simulink model "feedback_linearization_2015"  (R2020a)
settings: Solver=ode4  StartTime=0.0  StopTime=inf  FixedStep=0.002  RelTol=1e-3  EnableMultiTasking=on
undefined symbols (not defined in the file): Afe, g, gains_increasing, K, Kp_i_increasing, L, m, m0, REG_linearization, Ti_i_increasing, x, x_eq_increasing, y
libraries: PoliArd x6, simulink x6
settings Model: ExtModeTrigDuration=2  Creator=User  LastModifiedBy=miche
settings DataIOCC: LimitDataPoints=on  SaveFormat=Array  ReturnWorkspaceOutputs=off
settings OptimizationCC: LifeSpan=1  EfficientTunableParamExpr=on
settings DebuggingCC: UnderspecifiedInitializationDetection=Classic  MergeDetectMultiDrivingBlocksExec=none  SFUnexpectedBacktrackingDiag=warning  SFNoUnconditionalDefaultTransitionDiag=warning  SFExecutionAtInitializationDiag=none  ArithmeticOperatorsInVariantConditions=warning
settings HardwareCC: ProdBitPerPointer=32  ProdBitPerSizeT=32  ProdBitPerPtrDiffT=32  ProdLargestAtomicInteger=Long  ProdLargestAtomicFloat=Double  ProdIntDivRoundTo=Undefined  ProdWordSize=32  ProdHWDeviceType=ARM Compatible->ARM Cortex
settings ModelReferenceCC: PropagateSignalLabelsOutOfModel=off
settings SFSimCC: SimUseLocalCustomCode=off  MATLABDynamicMemAlloc=off  CustomCodeUndefinedFunction=UseInterfaceOnly
settings RTWCC: Description=Run on Target Hardware  SystemTargetFile=realtime.tlc  GenerateMakefile=off  TemplateMakefile=realtime.tmf  RTWVerbose=off  RTWUseLocalCustomCode=off
settings CodeAppCC: StateflowObjectComments=on
settings STFCustomTargetCC: TargetLibSuffix=.a  GenerateSampleERTMain=on  ERTCustomFileBanners=on  SupportNonInlinedSFcns=off  RemoveResetFunc=on  SupportVariableSizeSignals=on  MATLABClassNameForMDSCustomization=Simulink.SoftwareTarget.ERTCustomization  SystemTargetFile=realtime.tlc
settings ERTTargetCC: MultiwordLength=2048  GenerateSampleERTMain=on  ParMdlRefBuildCompliant=off  CompOptLevelCompliant=off  ConcurrentExecutionCompliant=off  CombineOutputUpdateFcns=off  SupportContinuousTime=on  SupportVariableSizeSignals=on  ModelStepFunctionPrototypeControlCompliant=off  CPPClassGenCompliant=off  UseToolchainInfoCompliant=off  ExtModeTransport=3  ExtModeMexFile=ext_serial_win32_comm_rtt  ExtModeMexArgs=0 1 9600  ERTSrcFileBannerTemplate=realtime_code_template.cgt  ERTHdrFileBannerTemplate=realtime_code_template.cgt  ERTDataSrcFileTemplate=realtime_code_template.cgt  ERTDataHdrFileTemplate=realtime_code_template.cgt  ERTCustomFileTemplate=realtime_file_process.tlc  ConvertIfToSwitch=off  SuppressUnreachableDefaultCases=off
settings ConfigComp: CovMetricSettings=dw  CovSaveCumulativeToWorkspaceVar=on  CovSaveSingleToWorkspaceVar=on  CovExternalEMLEnable=off

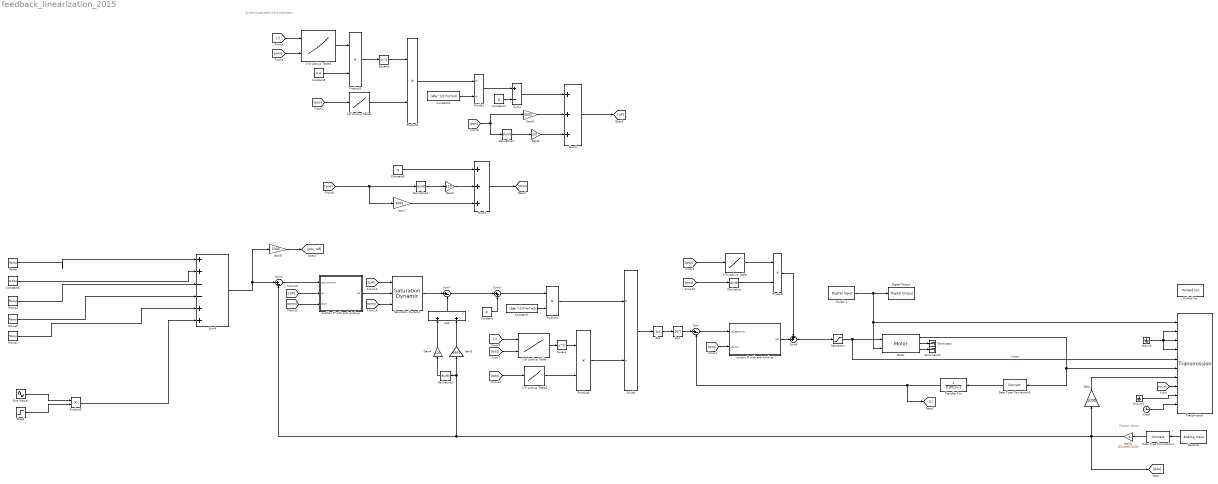
== system feedback_linearization_2015 ==
  note: Dynamic saturation limit estimation
  note: Position sensor
  1-D Lookup Table : Lookup_n-D  NumberOfTableDimensions=1  BreakpointsForDimension1=[0.0085 x_eq_increasing]  Table=[gains_increasing(1) gains_increasing]  InternalRulePriority=Speed  RndMeth=Simplest  InputSameDT=on
  1-D Lookup Table1 : Lookup_n-D  NumberOfTableDimensions=1  BreakpointsForDimension1=x  Table=K  InternalRulePriority=Speed  RndMeth=Simplest  InputSameDT=on
  1-D Lookup Table2 : Lookup_n-D  NumberOfTableDimensions=1  BreakpointsForDimension1=x  Table=K  InternalRulePriority=Speed  RndMeth=Simplest  InputSameDT=on
  2-D Lookup Table : Lookup_n-D  BreakpointsForDimension1=y  BreakpointsForDimension2=x  Table=L  InternalRulePriority=Speed  RndMeth=Simplest  InputSameDT=on
  2-D Lookup Table1 : Lookup_n-D  BreakpointsForDimension1=y  BreakpointsForDimension2=x  Table=L  InternalRulePriority=Speed  RndMeth=Simplest  InputSameDT=on
  Abs : Abs
  Add : Sum
  Clock : Clock
  Constant : Constant  Value=g
  Constant1 : Constant  Value=(Afe^(2))*m*m0
  Constant2 : Constant  Value=4.4
  Constant3 : Constant  Value=(Afe^(2))*m*m0
  Constant4 : Constant  Value=g
  Constant5 : Constant  Value=-g
  Constant6 : Constant  Value=0.014
  Data Type Conversion1 : DataTypeConversion
  Data Type Conversion5 : DataTypeConversion
  Derivative{,1..3} (4 alike) : Derivative
  Digital Output : PoliArd/Digital Output  DO_pin=1
  Divide : Product  Inputs=*/
  Divide1 : Product  Inputs=*/
  Gain : Gain  Gain=1000
  Gain1 : Gain  Gain=(20/4095)/1000
  Gain3 : Gain  Gain=3600
  Gain4 : Gain  Gain=120
  Gain5 : Gain  Gain=3600
  Gain6 : Gain  Gain=120
  Gain7 : Gain  Gain=3600
  Gain8 : Gain  Gain=120
  Gain9 : Gain  Gain=1000
  Ground : Ground
  Ground1 : Ground
  Motor : PoliArd/Motor  MotorID=2  DC_bus_mask=24  dt_mot=-1
  PoliArd Init : PoliArd/PoliArd Init
  Product{,1..5} (6 alike) : Product
  Ramp : simulink/Sources/Ramp  slope=0.001  start=7  InitialOutput=0
  Ramp1 : simulink/Sources/Ramp  slope=0.001  start=19  InitialOutput=0
  Ramp2 : simulink/Sources/Ramp  slope=0.001  start=17  InitialOutput=0
  Ramp3 : simulink/Sources/Ramp  slope=0.001  start=12  InitialOutput=0
  Saturation : Saturate  UpperLimit=18  LowerLimit=0
  Saturation Dynamic : simulink/Discontinuities/Saturation Dynamic  OutMin=[]  OutMax=[]  OutDataTypeStr=Inherit: Same as second input  OutDataType=fixdt(1, 16)  OutScaling=2^-10  DoSatur=off
  Sensore : PoliArd/Analog Input  AIpin_mask=2  AIsample=-1
  Sine Wave1 : Sin  Amplitude=0.002  Phase=0.3  SampleTime=0
  Sqrt : Sqrt  SaturateOnIntegerOverflow=on
  Square : Math  Operator=square  SignedPower=on  SaturateOnIntegerOverflow=on
  Square1 : Math  Operator=square  SignedPower=on  SaturateOnIntegerOverflow=on
  Step6 : Step  Time=28  SampleTime=0
  Sum : Sum  Inputs=|+-
  Sum1 : Sum  Inputs=|+-
  Sum2 : Sum  Inputs=+-
  Sum3 : Sum  Inputs=+++
  Sum4 : Sum  Inputs=+++
  Sum5 : Sum  Inputs=|++
  Sum6 : Sum  Inputs=|++--++
  Sum7 : Sum  Inputs=|+-
  Sum8 : Sum  Inputs=++|
  Switch 2 : PoliArd/Digital Input  DI_pin=2  DIsample=-1
  Terminator : Terminator
  Terminator1 : Terminator
  Transfer Fcn : TransferFcn  Denominator=[0.001 1]
  Transmission : PoliArd/Transmission  sample_freq=500  sig_to_send=6
  current PI with anti wind-up : Subsystem
      mask Display: disp('Current controller\n(PI)\nwith anti wind-up')
  position PI with anti wind-up : Subsystem
      mask Display: disp('Position controller\n(PI)\nwith anti wind-up')
  wires:
  Switch 2/1 -> Digital Output/1, Transmission/1, Motor/2
  Sensore/1 -> Data Type Conversion1/1
  Ground/1 -> Transmission/2, Transmission/4, Transmission/3
  Motor/1 -> Data Type Conversion5/1, Transmission/6
  Data Type Conversion1/1 -> Gain1/1
  Gain/1 -> Transmission/7
  Constant1/1 -> Product1/2
  Sum7/1 -> Sum5/1
  2-D Lookup Table/1 -> Square/1
  1-D Lookup Table1/1 -> Product2/2
  current PI with anti wind-up/1(out) -> Sum8/2
  Sum/1 -> current PI with anti wind-up/1(voltage error)
  Product/1 -> Sum8/1
  2-D Lookup Table1/1 -> Product3/1
  [UP] -> position PI with anti wind-up/2(up)
  Constant3/1 -> Divide1/2
  [pos] -> Derivative1/1, Gain5/1
  1-D Lookup Table2/1 -> Product4/2
  Gain5/1 -> Sum4/2
  Transfer Fcn/1 -> [i], Sum/2
  [pos] -> Derivative2/1, Gain7/1
  [i] -> 2-D Lookup Table1/1
  Gain4/1 -> Add/1
  [pos] -> current PI with anti wind-up/2(position)
  [i] -> 2-D Lookup Table/1
  Gain1/1 -> Derivative3/1, Gain3/1, Sum1/2, [pos], Gain/1
  Sum2/1 -> Sum4/1
  Abs/1 -> Sqrt/1
  [pos] -> 2-D Lookup Table1/2
  position PI with anti wind-up/1(out) -> Saturation Dynamic/2
  Sum3/1 -> [DOWN]
  [UP] -> Saturation Dynamic/1
  1-D Lookup Table/1 -> Product/1
  Derivative3/1 -> Gain4/1
  [pos] -> 1-D Lookup Table/1
  Sum1/1 -> position PI with anti wind-up/1(position error)
  Square1/1 -> Product2/1
  Product3/1 -> Square1/1
  Gain3/1 -> Add/2
  [pos] -> 1-D Lookup Table2/1
  Constant4/1 -> Sum2/2
  Product2/1 -> Divide1/1
  Gain8/1 -> Sum3/2
  Derivative1/1 -> Gain6/1
  Product4/1 -> Divide/2
  Gain7/1 -> Sum3/3
  Product1/1 -> Divide/1
  Sqrt/1 -> Sum/1
  Constant2/1 -> Product3/2
  Square/1 -> Product4/1
  [DOWN] -> position PI with anti wind-up/3(down)
  Saturation/1 -> Transmission/5, Motor/1  "voltage"
  Divide/1 -> Abs/1
  Gain6/1 -> Sum4/3
  Sum5/1 -> Product1/1
  [pos] -> 1-D Lookup Table1/1
  Saturation Dynamic/1 -> Sum7/1
  Sum4/1 -> [UP]
  [DOWN] -> Saturation Dynamic/3
  Derivative/1 -> Product/2
  Constant/1 -> Sum5/2
  Divide1/1 -> Sum2/1
  Derivative2/1 -> Gain8/1
  [pos] -> 2-D Lookup Table/2
  Constant5/1 -> Sum3/1
  Sum8/1 -> Saturation/1
  Add/1 -> Sum7/2
  [pos] -> Derivative/1
  Data Type Conversion5/1 -> Transfer Fcn/1
  Motor/2 -> Terminator/1
  Motor/3 -> Terminator1/1
  [pos_ref] -> Transmission/8
  Ground1/1 -> Transmission/9
  Gain9/1 -> [pos_ref]
  Clock/1 -> Transmission/10
  Ramp/1 -> Sum6/1
  Constant6/1 -> Sum6/2
  Ramp3/1 -> Sum6/3
  Ramp2/1 -> Sum6/4
  Ramp1/1 -> Sum6/5
  Sine Wave1/1 -> Product5/1
  Step6/1 -> Product5/2
  Product5/1 -> Sum6/6
  Sum6/1 -> Gain9/1, Sum1/1

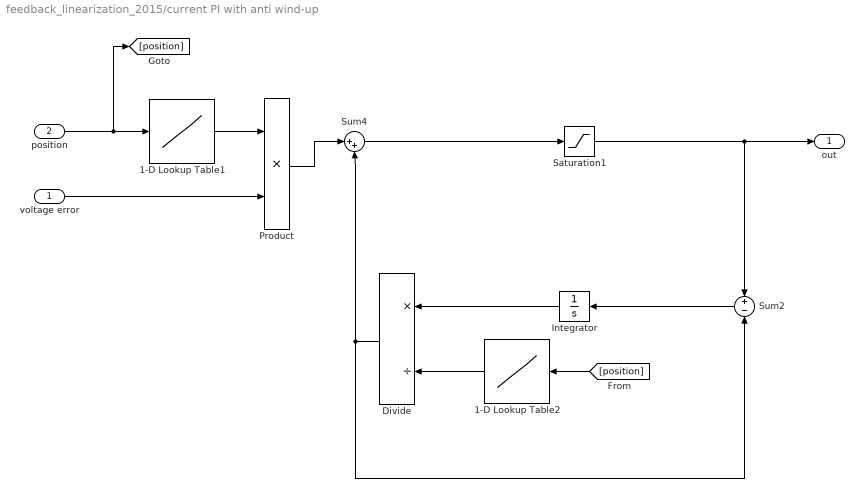
== system feedback_linearization_2015/current PI with anti wind-up ==
  voltage error : Inport
  position : Inport  Port=2
  1-D Lookup Table1 : Lookup_n-D  NumberOfTableDimensions=1  BreakpointsForDimension1=[0.0085 x_eq_increasing]  Table=[Kp_i_increasing(1) Kp_i_increasing]  InternalRulePriority=Speed  RndMeth=Simplest  InputSameDT=on
  1-D Lookup Table2 : Lookup_n-D  NumberOfTableDimensions=1  BreakpointsForDimension1=[0.0085 x_eq_increasing]  Table=[Ti_i_increasing(1) Ti_i_increasing]  InternalRulePriority=Speed  RndMeth=Simplest  InputSameDT=on
  Divide : Product  Inputs=*/
  Integrator : Integrator
  Product : Product
  Saturation1 : Saturate  UpperLimit=18  LowerLimit=0
  Sum2 : Sum  Inputs=+|-
  Sum4 : Sum  Inputs=|++
  out : Outport
  wires:
  Sum4/1 -> Saturation1/1
  Product/1 -> Sum4/1
  Saturation1/1 -> out/1, Sum2/1
  voltage error/1 -> Product/2
  1-D Lookup Table1/1 -> Product/1
  position/1 -> [position], 1-D Lookup Table1/1
  Divide/1 -> Sum2/2, Sum4/2
  Sum2/1 -> Integrator/1
  Integrator/1 -> Divide/1
  1-D Lookup Table2/1 -> Divide/2
  [position] -> 1-D Lookup Table2/1

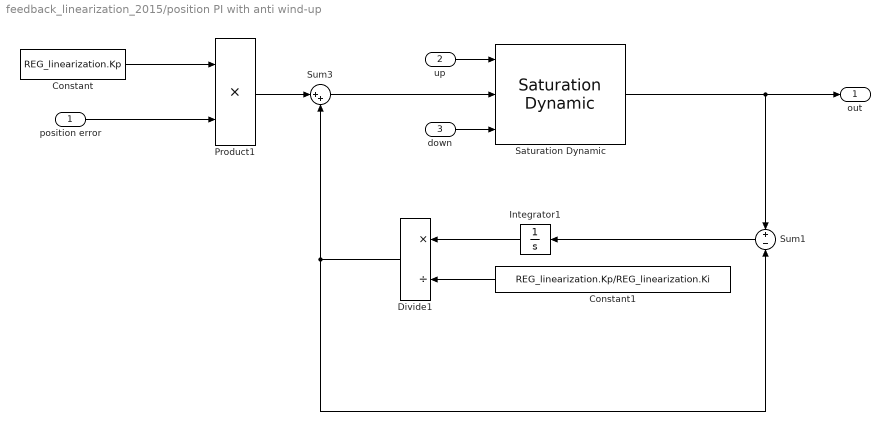
== system feedback_linearization_2015/position PI with anti wind-up ==
  position error : Inport
  up : Inport  Port=2
  down : Inport  Port=3
  Constant : Constant  Value=REG_linearization.Kp
  Constant1 : Constant  Value=REG_linearization.Kp/REG_linearization.Ki
  Divide1 : Product  Inputs=*/
  Integrator1 : Integrator
  Product1 : Product
  Saturation Dynamic : simulink/Discontinuities/Saturation Dynamic  OutMin=[]  OutMax=[]  OutDataTypeStr=Inherit: Same as second input  OutDataType=fixdt(1, 16)  OutScaling=2^-10  DoSatur=off
  Sum1 : Sum  Inputs=+|-
  Sum3 : Sum  Inputs=|++
  out : Outport
  wires:
  Sum1/1 -> Integrator1/1
  Divide1/1 -> Sum1/2, Sum3/2
  Product1/1 -> Sum3/1
  position error/1 -> Product1/2
  Constant/1 -> Product1/1
  Constant1/1 -> Divide1/2
  Integrator1/1 -> Divide1/1
  Saturation Dynamic/1 -> out/1, Sum1/1
  Sum3/1 -> Saturation Dynamic/2
  down/1 -> Saturation Dynamic/3
  up/1 -> Saturation Dynamic/1
